simulink model "Q1"  (R2020b)
settings: Solver=VariableStepAuto  StartTime=0.0  StopTime=10  RelTol=1e-3
settings Model: Creator=asus  LastModifiedBy=asus

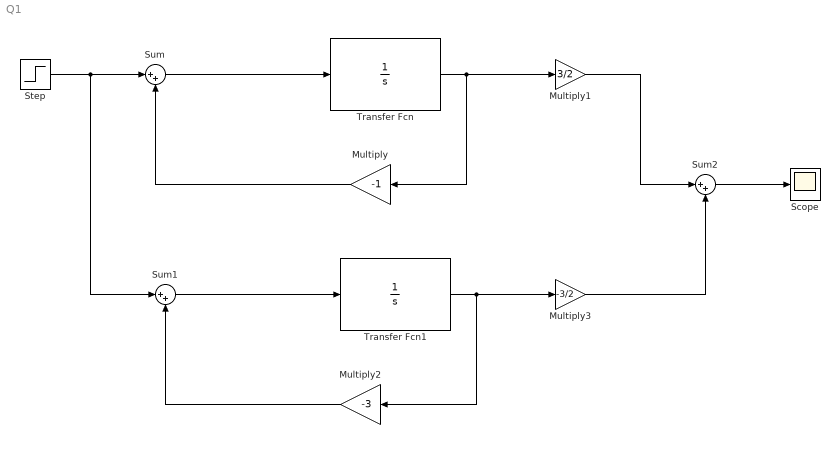
== system Q1 ==
  Multiply : Gain  Gain=-1
  Multiply1 : Gain  Gain=3/2
  Multiply2 : Gain  Gain=-3
  Multiply3 : Gain  Gain=-3/2
  Scope : Scope
  Step : Step  Time=0.001  SampleTime=0
  Sum : Sum  Inputs=|++
  Sum1 : Sum  Inputs=|++
  Sum2 : Sum  Inputs=|++
  Transfer Fcn : TransferFcn  Denominator=[1 0]
  Transfer Fcn1 : TransferFcn  Denominator=[1 0]
  wires:
  Transfer Fcn/1 -> Multiply/1, Multiply1/1
  Multiply/1 -> Sum/2
  Sum/1 -> Transfer Fcn/1
  Sum1/1 -> Transfer Fcn1/1
  Transfer Fcn1/1 -> Multiply2/1, Multiply3/1
  Step/1 -> Sum1/1, Sum/1
  Multiply2/1 -> Sum1/2
  Multiply1/1 -> Sum2/1
  Multiply3/1 -> Sum2/2
  Sum2/1 -> Scope/1
